simulink model "Stepper_motor"  (R2022a)
settings: Solver=VariableStepAuto  StartTime=0.0  StopTime=20  RelTol=1e-3
undefined symbols (not defined in the file): out
libraries: spsIdealSwitchLib x4, spsDCVoltageSourceLib x1, spsStepperMotorLib x1, spspowerguiLib x1
settings Model: Creator=Admin  LastModifiedBy=Admin
settings SolverCC: MaxZcPerStep=1

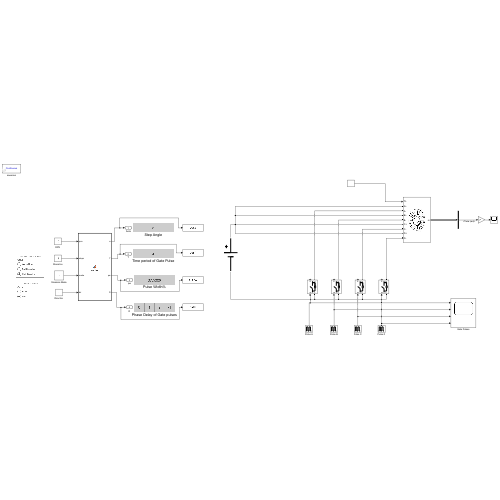
[thumbnail: Simulink's stored preview of the top-level diagram]
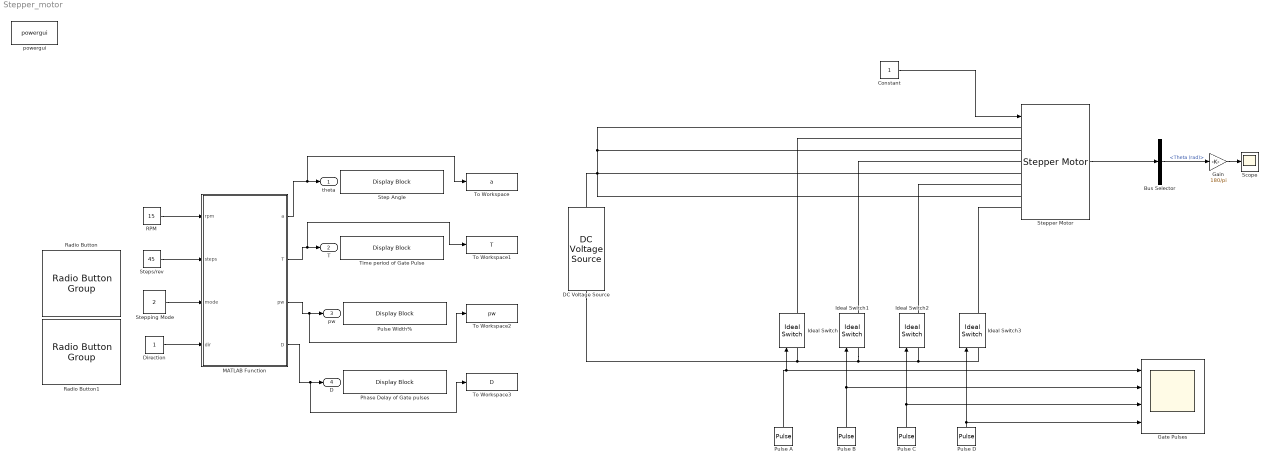
== system Stepper_motor ==
  Bus Selector : BusSelector  OutputSignals=Theta (rad)
  Constant : Constant
  DC Voltage Source : spsDCVoltageSourceLib/DC Voltage Source  Amplitude=25  Measurements=None
  Direction : Constant
  Gain : Gain  Gain=180/pi
  Gate Pulses : Scope  NumInputPorts=4
  Ideal Switch{,1..3} (4 alike) : spsIdealSwitchLib/Ideal Switch  Ron=0.001  Lon=0  IC=0  Rs=1e5  Cs=inf  Measurements=on
  MATLAB Function : MATLAB Function  TreatAsAtomicUnit=on
  Phase Delay of Gate pulses : DisplayBlock  LabelPosition=Hide  Transparency=1
  Pulse A : DiscretePulseGenerator  PulseType=Time based  Amplitude=5  Period=out.T.signals.values(1,1)  PulseWidth=out.pw.signals.values(1,1)  PhaseDelay=out.D.signals.values(1,1,1)
  Pulse B : DiscretePulseGenerator  PulseType=Time based  Amplitude=5  Period=out.T.signals.values(1,1)  PulseWidth=out.pw.signals.values(1,1)  PhaseDelay=out.D.signals.values(1,2,1)
  Pulse C : DiscretePulseGenerator  PulseType=Time based  Amplitude=5  Period=out.T.signals.values(1,1)  PulseWidth=out.pw.signals.values(1,1)  PhaseDelay=out.D.signals.values(1,3,1)
  Pulse D : DiscretePulseGenerator  PulseType=Time based  Amplitude=5  Period=out.T.signals.values(1,1)  PulseWidth=out.pw.signals.values(1,1)  PhaseDelay=out.D.signals.values(1,4,1)
  Pulse Width% : DisplayBlock  LabelPosition=Hide  Transparency=1
  RPM : Constant  Value=15
  Radio Button : RadioButtonGroup  SelectedLabel=Half Stepping  ButtonGroupName=Group
      settings: Values={{'Wave Drive', 'Full Stepping', 'Half Stepping'}, [0 1 2]}
  Radio Button1 : RadioButtonGroup  SelectedLabel=CW  ButtonGroupName=Group
      settings: Values={{'ACW', 'CW'}, [-1 1]}
  Scope : Scope
  Step Angle : DisplayBlock  LabelPosition=Hide  Transparency=1
  Stepper Motor : spsStepperMotorLib/Stepper Motor  MotorType=Variable reluctance  NumberOfPhases_1=2  NumberOfPhases_2=4  PresetModel_1=<empty>  PresetModel_2=<empty>  L=10e-3  Lmax=10e-3  Lmin=2e-3  R=1.2  Step_angle=30  Psim=0.04  Tdm=0.02  J=1e-4/5  B=1e-3  w0=0  pos0=60  TsPowergui=0  TsBlock=-1
      settings: SourceProductBaseCode=PS
  Stepping Mode : Constant  Value=2  SampleTime=-1
  Steps/rev : Constant  Value=45
  Time period of Gate Pulse : DisplayBlock  LabelPosition=Hide  Transparency=1
  To Workspace : ToWorkspace  VariableName=a  SaveFormat=Structure  SampleTime=-1
      settings: Save2DSignal=2-D array (concatenate along first dimension)
  To Workspace1 : ToWorkspace  VariableName=T  SaveFormat=Structure  SampleTime=-1
      settings: Save2DSignal=2-D array (concatenate along first dimension)
  To Workspace2 : ToWorkspace  VariableName=pw  SaveFormat=Structure  SampleTime=-1
      settings: Save2DSignal=2-D array (concatenate along first dimension)
  To Workspace3 : ToWorkspace  VariableName=D  SaveFormat=Structure  SampleTime=-1
      settings: Save2DSignal=2-D array (concatenate along first dimension)
  powergui : spspowerguiLib/powergui  Priority=1  SimulationMode=Continuous  SampleTime=50e-6  frequency=60  Iterations=50  frequencyindice=0  Pbase=100e6  ErrMax=1e-4  UnitsV=kV  UnitsW=MW  buscounter=0  FunctionMessages=off  echomessages=off  EnableUseOfTLC=off  CurrentSourceSwitches=off  DisableSnubberDevices=off  DisableRonSwitches=off  DisableVfSwitches=off  DisplayEquations=off  AutomaticDiscreteSolvers=off  SolverType=Tustin/Backward Euler (TBE)  Interpol=off  ExternalGateDelay=off  methode=off  Ts=100  x0status=blocks  SPID=on  SwTol=0  HookPort=off  NonlinearTolerance=1e-4  nMaxIteration=100  ContinueOnMaxIteration=off  RestoreLinks=warning  ResistiveCurrentMeasurement=off  Frange=[0:2:500]  Ylog=off  Xlog=on  ShowGrid=off  save=off  variable=ZData  structure=0  ZoomFFT=off  StartTime=0.0  cycles=1  DisplayStyle=1  fundamental=60  FreqAxis=off  MaxFrequency=1000  frequencyindicesteady=1  RmsSteady=1  display=off
  theta : Outport
  T : Outport  Port=2
  pw : Outport  Port=3
  D : Outport  Port=4
  wires:
  Stepping Mode/1 -> MATLAB Function/3(mode)
  MATLAB Function/2(T) -> To Workspace1/1, T/1
  RPM/1 -> MATLAB Function/1(rpm)
  Direction/1 -> MATLAB Function/4(dir)
  Steps/rev/1 -> MATLAB Function/2(steps)
  MATLAB Function/4(D) -> To Workspace3/1, D/1
  MATLAB Function/1(a) -> To Workspace/1, theta/1
  MATLAB Function/3(pw) -> To Workspace2/1, pw/1
  Pulse A/1 -> Gate Pulses/1, Ideal Switch/1
  Pulse C/1 -> Gate Pulses/3, Ideal Switch2/1
  Pulse D/1 -> Gate Pulses/4, Ideal Switch3/1
  Pulse B/1 -> Gate Pulses/2, Ideal Switch1/1
  Stepper Motor/1 -> Bus Selector/1
  Bus Selector/1 -> Gain/1  "<Theta (rad)>"
  Gain/1 -> Scope/1
  Constant/1 -> Stepper Motor/1
  connections:
  Ideal Switch2/LConn1 -- Ideal Switch3/LConn1 -- DC Voltage Source/LConn1 -- Ideal Switch/LConn1 -- Ideal Switch1/LConn1
  Stepper Motor/LConn1 -- Stepper Motor/LConn3 -- DC Voltage Source/RConn1 -- Stepper Motor/LConn7 -- Stepper Motor/LConn5
  Ideal Switch/RConn1 -- Stepper Motor/LConn2
  Ideal Switch1/RConn1 -- Stepper Motor/LConn4
  Ideal Switch2/RConn1 -- Stepper Motor/LConn6
  Ideal Switch3/RConn1 -- Stepper Motor/LConn8

== matlab function Stepper_motor/MATLAB Function ==
  data: rpm input; steps input; mode input; dir input; a output; T output; pw output; D output
function [a,T, pw, D] = control (rpm, steps, mode, dir)

D = zeros(1,4);
w = 0;

T = 60/rpm;


if mode == 0
    w = 25;
end
if mode == 1
    w = 50;
end
if mode == 2
    w = 37.5;
end


if dir == 1
    D(2) = T/4;
    D(3) = T/2;
    D(4) = -T/4;

else 
    D(2) = -T/4;
    D(3) = T/2;
    D(4) = T/4;
end

a = 360/steps;
T = 60/rpm;
pw = w;
end
